simulink model "plataforma_unlp_GSAFE_v2"  (R2016b)
settings: Solver=ode1  StartTime=escenario.ti  StopTime=escenario.tf  FixedStep=escenario.paso  RelTol=1e-3  EnableMultiTasking=on
undefined symbols (not defined in the file): ctrl, escenario, hardware, lazo, lazoh, parametros, PDB_IFB_GSAFE_v2, settings
settings Model: Creator=Administrador  LastModifiedBy=Nicolas
settings DataIOCC: SaveFormat=Array  SaveState=on  StateSaveName=estados  OutputSaveName=salidas
settings OptimizationCC: ExpressionDepthLimit=2147483647  LifeSpan=inf
settings DebuggingCC: UnderspecifiedInitializationDetection=Classic  MergeDetectMultiDrivingBlocksExec=none  SolverPrmCheckMsg=warning  StateNameClashWarn=warning  SFUnexpectedBacktrackingDiag=warning  SFNoUnconditionalDefaultTransitionDiag=warning  SFExecutionAtInitializationDiag=none
settings HardwareCC: ProdBitPerPointer=32  ProdBitPerSizeT=32  ProdBitPerPtrDiffT=32  ProdLargestAtomicFloat=None  ProdIntDivRoundTo=Undefined  ProdEndianess=Unspecified  ProdWordSize=32  ProdHWDeviceType=32-bit Generic
settings ModelReferenceCC: PropagateSignalLabelsOutOfModel=off
settings GRTTargetCC: TargetLangStandard=C89/C90 (ANSI)  GeneratePreprocessorConditionals=Disable all
settings ConfigComp: CovMetricSettings=dw  CovHtmlReporting=on  CovSaveCumulativeToWorkspaceVar=on  CovSaveSingleToWorkspaceVar=on  CovExternalEMLEnable=off

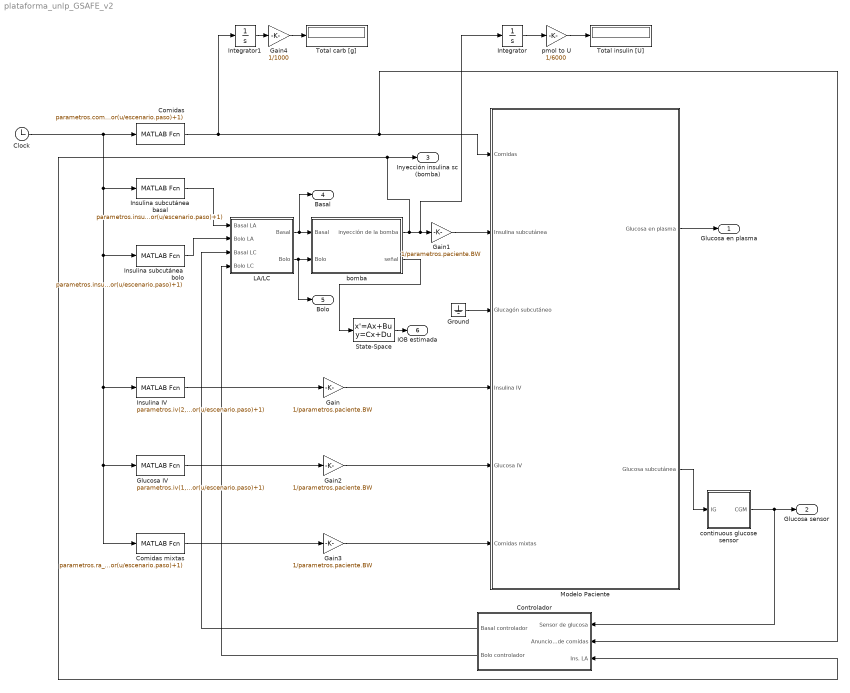
== system plataforma_unlp_GSAFE_v2 ==
  Clock : Clock
  Comidas : MATLABFcn  MATLABFcn=parametros.comidas(1,floor(u/escenario.paso)+1)  OutputDimensions=1  OutputSignalType=real  Output1D=off
  Comidas mixtas : MATLABFcn  MATLABFcn=parametros.ra_comidas_mixtas(1,floor(u/escenario.paso)+1)  OutputDimensions=1  OutputSignalType=real  Output1D=off
  Controlador : Subsystem
  Gain{,1..3} (4 alike) : Gain  Gain=1/parametros.paciente.BW
  Gain4 : Gain  Gain=1/1000
  Glucosa IV : MATLABFcn  MATLABFcn=parametros.iv(1,floor(u/escenario.paso)+1)  OutputDimensions=1  OutputSignalType=real  Output1D=off
  Ground : Ground
  Insulina IV : MATLABFcn  MATLABFcn=parametros.iv(2,floor(u/escenario.paso)+1)  OutputDimensions=1  OutputSignalType=real  Output1D=off
  Insulina subcutánea basal : MATLABFcn  MATLABFcn=parametros.insulina(2,floor(u/escenario.paso)+1)  OutputDimensions=1  OutputSignalType=real  Output1D=off
  Insulina subcutánea bolo : MATLABFcn  MATLABFcn=parametros.insulina(1,floor(u/escenario.paso)+1)  OutputDimensions=1  OutputSignalType=real  Output1D=off
  Integrator : Integrator
  Integrator1 : Integrator
  LA/LC : Subsystem
  Modelo Paciente : Subsystem
  State-Space : StateSpace  A=[-ctrl.KDIA 0;ctrl.KDIA -ctrl.KDIA]  B=[1/6000;0]  C=[1 1]  D=0  X0=[ctrl.Iee/ctrl.KDIA/6000;ctrl.Iee/ctrl.KDIA/6000]
  Total carb [g] : Display
  Total insulin [U] : Display
  bomba : Subsystem
  continuous glucose sensor : Subsystem
  pmol to U : Gain  Gain=1/6000
  Glucosa en plasma : Outport
  Glucosa sensor : Outport  Port=2
  Inyección insulina sc (bomba) : Outport  Port=3
  Basal : Outport  Port=4
  Bolo : Outport  Port=5
  IOB estimada : Outport  Port=6
  wires:
  Insulina IV/1 -> Gain/1
  Gain/1 -> Modelo Paciente/4(Insulina IV)
  Gain1/1 -> Modelo Paciente/2(Insulina subcutánea)
  Glucosa IV/1 -> Gain2/1
  Gain2/1 -> Modelo Paciente/5(Glucosa IV)
  Comidas/1 -> Integrator1/1, Controlador/2(Anuncio de comidas), Modelo Paciente/1(Comidas)
  Comidas mixtas/1 -> Gain3/1
  Gain3/1 -> Modelo Paciente/6(Comidas mixtas)
  Modelo Paciente/2(Glucosa subcutánea) -> continuous glucose sensor/1(IG)
  continuous glucose sensor/1(CGM) -> Glucosa sensor/1, Controlador/1(Sensor de glucosa)
  bomba/1(inyección de la bomba) -> Controlador/3(Ins. LA), Inyección insulina sc (bomba)/1, Integrator/1, Gain1/1
  bomba/2(señal) -> State-Space/1
  Insulina subcutánea basal/1 -> LA/LC/1(Basal LA)
  Insulina subcutánea bolo/1 -> LA/LC/2(Bolo LA)
  Controlador/1(Basal controlador) -> LA/LC/3(Basal LC)
  Controlador/2(Bolo controlador) -> LA/LC/4(Bolo LC)
  LA/LC/1(Basal) -> Basal/1, bomba/1(Basal)
  LA/LC/2(Bolo) -> bomba/2(Bolo), Bolo/1
  Integrator1/1 -> Gain4/1
  Gain4/1 -> Total carb [g]/1
  Integrator/1 -> pmol to U/1
  pmol to U/1 -> Total insulin [U]/1
  Clock/1 -> Comidas/1, Insulina subcutánea bolo/1, Comidas mixtas/1, Glucosa IV/1, Insulina IV/1, Insulina subcutánea basal/1
  State-Space/1 -> IOB estimada/1
  Modelo Paciente/1(Glucosa en plasma) -> Glucosa en plasma/1
  Ground/1 -> Modelo Paciente/3(Glucagón subcutáneo)

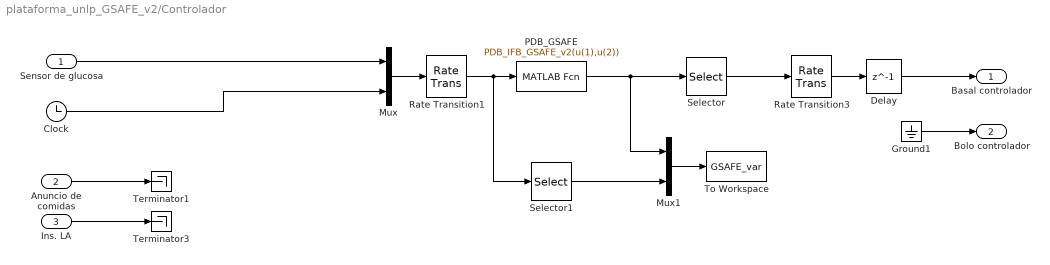
== system plataforma_unlp_GSAFE_v2/Controlador ==
  Sensor de glucosa : Inport
  Anuncio de comidas : Inport  Port=2
  Ins. LA : Inport  Port=3
  Clock : Clock
  Delay : Delay  DelayLength=1  InitialCondition=ctrl.Iee  SampleTime=ctrl.paso
  Ground1 : Ground
  Mux : Mux  Inputs=2
  Mux1 : Mux  Inputs=2
  PDB_GSAFE : MATLABFcn  MATLABFcn=PDB_IFB_GSAFE_v2(u(1),u(2))  OutputDimensions=2
  Rate Transition1 : RateTransition  OutPortSampleTime=ctrl.Ts
  Rate Transition3 : RateTransition  X0=ctrl.Iee  OutPortSampleTime=ctrl.paso
  Selector : Selector  InputPortWidth=2  IndexOptions=Index vector (dialog)  Indices=1  OutputSizes=1
  Selector1 : Selector  InputPortWidth=2  IndexOptions=Index vector (dialog)  Indices=1  OutputSizes=1
  Terminator1 : Terminator
  Terminator3 : Terminator
  To Workspace : ToWorkspace  VariableName=GSAFE_var  SampleTime=ctrl.Ts
  Basal controlador : Outport
  Bolo controlador : Outport  Port=2
  wires:
  Ins. LA/1 -> Terminator3/1
  Mux/1 -> Rate Transition1/1
  PDB_GSAFE/1 -> Mux1/1, Selector/1
  Ground1/1 -> Bolo controlador/1
  Rate Transition3/1 -> Delay/1
  Selector/1 -> Rate Transition3/1
  Mux1/1 -> To Workspace/1
  Sensor de glucosa/1 -> Mux/1
  Anuncio de comidas/1 -> Terminator1/1
  Rate Transition1/1 -> Selector1/1, PDB_GSAFE/1
  Clock/1 -> Mux/2
  Selector1/1 -> Mux1/2
  Delay/1 -> Basal controlador/1

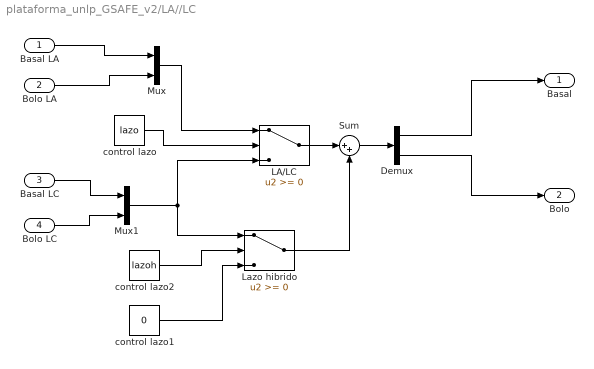
== system plataforma_unlp_GSAFE_v2/LA//LC ==
  Basal LA : Inport
  Bolo LA : Inport  Port=2
  Basal LC : Inport  Port=3
  Bolo LC : Inport  Port=4
  Demux : Demux  Outputs=2
  LA/LC : Switch
  Lazo hibrido : Switch
  Mux : Mux  Inputs=2
  Mux1 : Mux  Inputs=2
  Sum : Sum  Inputs=|++
  control lazo : Constant  Value=lazo
  control lazo1 : Constant  Value=0
  control lazo2 : Constant  Value=lazoh
  Basal : Outport
  Bolo : Outport  Port=2
  wires:
  Basal LA/1 -> Mux/1
  Bolo LA/1 -> Mux/2
  Basal LC/1 -> Mux1/1
  Bolo LC/1 -> Mux1/2
  Mux/1 -> LA/LC/1
  control lazo/1 -> LA/LC/2
  Mux1/1 -> LA/LC/3, Lazo hibrido/1
  Demux/1 -> Basal/1
  Demux/2 -> Bolo/1
  LA/LC/1 -> Sum/1
  Sum/1 -> Demux/1
  Lazo hibrido/1 -> Sum/2
  control lazo2/1 -> Lazo hibrido/2
  control lazo1/1 -> Lazo hibrido/3

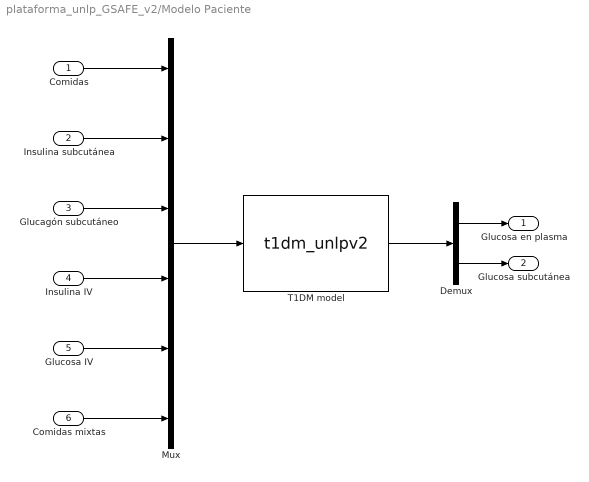
== system plataforma_unlp_GSAFE_v2/Modelo Paciente ==
  Comidas : Inport
  Insulina subcutánea : Inport  Port=2
  Glucagón subcutáneo : Inport  Port=3
  Insulina IV : Inport  Port=4
  Glucosa IV : Inport  Port=5
  Comidas mixtas : Inport  Port=6
  Demux : Demux  Outputs=2
  Mux : Mux  Inputs=6
  T1DM model : S-Function  FunctionName=t1dm_unlpv2  Parameters=parametros,escenario  SFunctionDeploymentMode=off  EnableBusSupport=off
  Glucosa en plasma : Outport
  Glucosa subcutánea : Outport  Port=2
  wires:
  Mux/1 -> T1DM model/1
  Insulina subcutánea/1 -> Mux/2
  Insulina IV/1 -> Mux/4
  Glucosa IV/1 -> Mux/5
  Comidas/1 -> Mux/1
  Comidas mixtas/1 -> Mux/6
  T1DM model/1 -> Demux/1
  Glucagón subcutáneo/1 -> Mux/3
  Demux/1 -> Glucosa en plasma/1
  Demux/2 -> Glucosa subcutánea/1

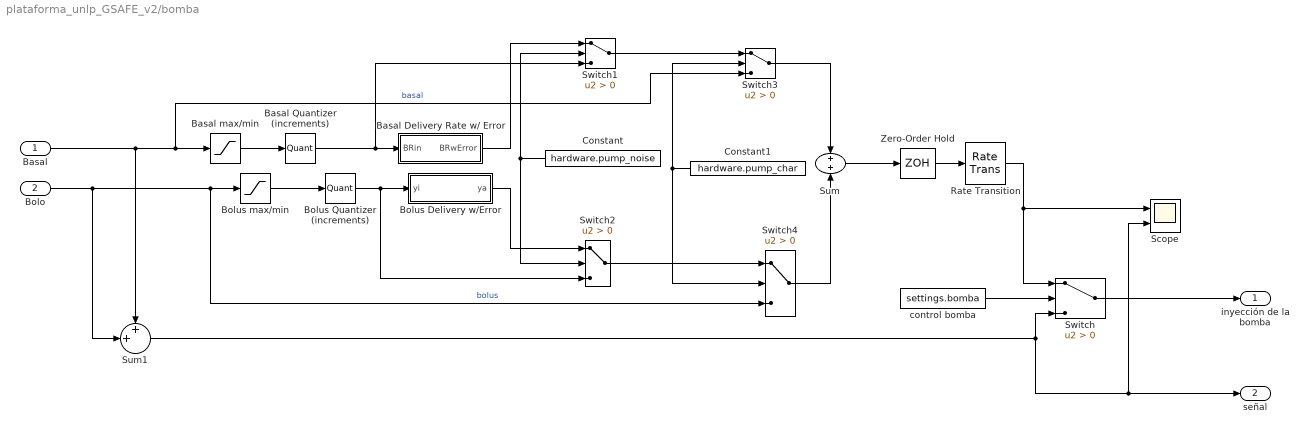
== system plataforma_unlp_GSAFE_v2/bomba ==
  Basal : Inport
  Bolo : Inport  Port=2
  Basal Delivery Rate w/ Error : Subsystem
  Basal Quantizer (increments) : Quantizer  QuantizationInterval=hardware.pump_basal_inc
  Basal max/min : Saturate  UpperLimit=hardware.pump_basal_max  LowerLimit=hardware.pump_basal_min
  Bolus Delivery w/Error : Subsystem
  Bolus Quantizer (increments) : Quantizer  QuantizationInterval=hardware.pump_bolus_inc
  Bolus max/min : Saturate  UpperLimit=hardware.pump_bolus_max  LowerLimit=0
  Constant : Constant  Value=hardware.pump_noise
  Constant1 : Constant  Value=hardware.pump_char
  Rate Transition : RateTransition
  Scope : Scope  NumInputPorts=2
  Sum : Sum  Inputs=+|+
  Sum1 : Sum  Inputs=++|
  Switch{,1..4} (5 alike) : Switch  Criteria=u2 > Threshold
  Zero-Order Hold : ZeroOrderHold  SampleTime=hardware.pump_sampling
  control bomba : Constant  Value=settings.bomba
  inyección de la bomba : Outport
  señal : Outport  Port=2
  wires:
  control bomba/1 -> Switch/2
  Switch/1 -> inyección de la bomba/1
  Sum1/1 -> Scope/2, señal/1, Switch/3
  Zero-Order Hold/1 -> Rate Transition/1
  Bolus max/min/1 -> Bolus Quantizer (increments)/1
  Sum/1 -> Zero-Order Hold/1
  Basal/1 -> Sum1/1, Basal max/min/1, Switch3/3  "basal"
  Basal max/min/1 -> Basal Quantizer (increments)/1
  Bolo/1 -> Sum1/2, Switch4/3, Bolus max/min/1  "bolus"
  Bolus Quantizer (increments)/1 -> Switch2/3, Bolus Delivery w/Error/1(yi)
  Basal Quantizer (increments)/1 -> Switch1/3, Basal Delivery Rate w/ Error/1(BRin)
  Basal Delivery Rate w/ Error/1(BRwError) -> Switch1/1
  Constant/1 -> Switch2/2, Switch1/2
  Bolus Delivery w/Error/1(ya) -> Switch2/1
  Switch2/1 -> Switch4/1
  Switch1/1 -> Switch3/1
  Constant1/1 -> Switch4/2, Switch3/2
  Switch3/1 -> Sum/1
  Switch4/1 -> Sum/2
  Rate Transition/1 -> Scope/1, Switch/1

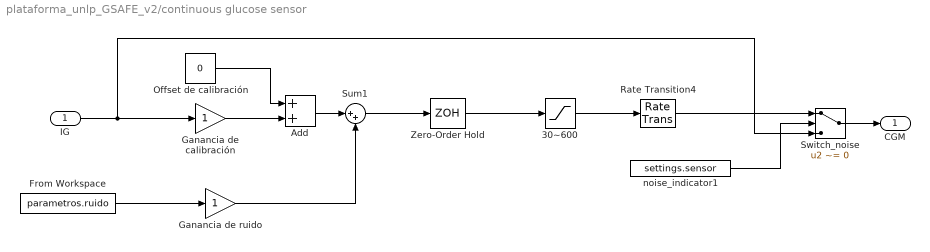
== system plataforma_unlp_GSAFE_v2/continuous glucose sensor ==
  IG : Inport
  30~600 : Saturate  UpperLimit=hardware.sensor_max  LowerLimit=hardware.sensor_min
  Add : Sum
  From Workspace : FromWorkspace  VariableName=parametros.ruido  SampleTime=0
  Ganancia de calibración : Gain
  Ganancia de ruido : Gain
  Offset de calibración : Constant  Value=0
  Rate Transition4 : RateTransition  X0=parametros.paciente.x0(4)/parametros.paciente.Vg  OutPortSampleTime=escenario.paso
  Sum1 : Sum  Inputs=|++
  Switch_noise : Switch  Criteria=u2 ~= 0  Threshold=1440
  Zero-Order Hold : ZeroOrderHold  SampleTime=hardware.sensor_sampling
  noise_indicator1 : Constant  Value=settings.sensor
  CGM : Outport
  wires:
  Sum1/1 -> Zero-Order Hold/1
  Zero-Order Hold/1 -> 30~600/1
  30~600/1 -> Rate Transition4/1
  Offset de calibración/1 -> Add/1
  Ganancia de calibración/1 -> Add/2
  Add/1 -> Sum1/1
  Rate Transition4/1 -> Switch_noise/1
  noise_indicator1/1 -> Switch_noise/2
  IG/1 -> Switch_noise/3, Ganancia de calibración/1
  Switch_noise/1 -> CGM/1
  From Workspace/1 -> Ganancia de ruido/1
  Ganancia de ruido/1 -> Sum1/2

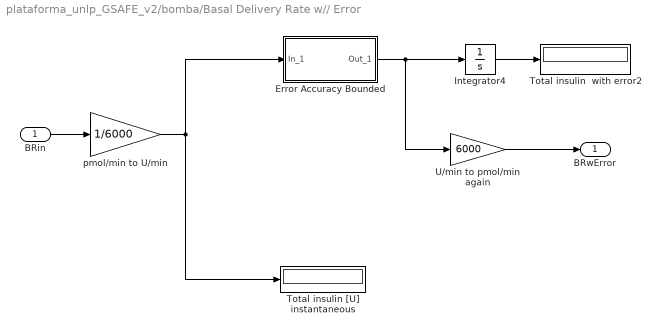
== system plataforma_unlp_GSAFE_v2/bomba/Basal Delivery Rate w// Error ==
  BRin : Inport
  Error Accuracy Bounded : Subsystem
  Integrator4 : Integrator
  Total insulin  with error2 : Display
  Total insulin [U] instantaneous : Display
  U/min to pmol/min again : Gain  Gain=6000
  pmol/min to U/min : Gain  Gain=1/6000
  BRwError : Outport
  wires:
  Integrator4/1 -> Total insulin  with error2/1
  Error Accuracy Bounded/1(Out_1) -> Integrator4/1, U/min to pmol/min again/1
  U/min to pmol/min again/1 -> BRwError/1
  pmol/min to U/min/1 -> Error Accuracy Bounded/1(In_1), Total insulin [U] instantaneous/1
  BRin/1 -> pmol/min to U/min/1

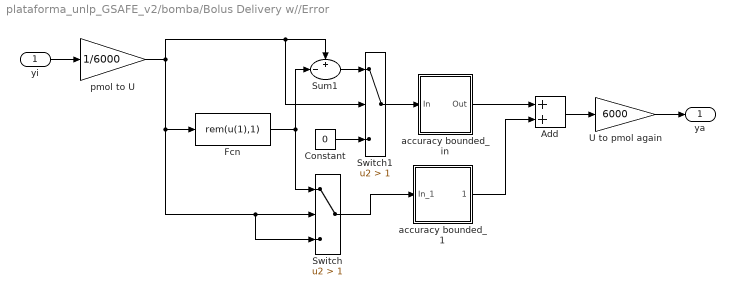
== system plataforma_unlp_GSAFE_v2/bomba/Bolus Delivery w//Error ==
  yi : Inport
  Add : Sum
  Constant : Constant  Value=0
  Fcn : Fcn  Expr=rem(u(1),1)
  Sum1 : Sum  Inputs=+-|
  Switch : Switch  Criteria=u2 > Threshold  Threshold=1
  Switch1 : Switch  Criteria=u2 > Threshold  Threshold=1
  U to pmol again : Gain  Gain=6000
  accuracy bounded_1 : Subsystem
  accuracy bounded_in : Subsystem
  pmol to U : Gain  Gain=1/6000
  ya : Outport
  wires:
  Switch1/1 -> accuracy bounded_in/1(In)
  Constant/1 -> Switch1/3
  Sum1/1 -> Switch1/1
  Switch/1 -> accuracy bounded_1/1(In_1)
  Fcn/1 -> Sum1/2, Switch/1
  accuracy bounded_1/1(Out_1) -> Add/2
  accuracy bounded_in/1(Out) -> Add/1
  Add/1 -> U to pmol again/1
  U to pmol again/1 -> ya/1
  pmol to U/1 -> Switch1/2, Sum1/1, Switch/3, Switch/2, Fcn/1
  yi/1 -> pmol to U/1

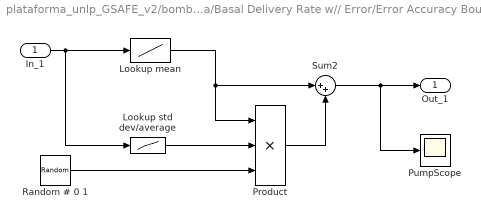
== system plataforma_unlp_GSAFE_v2/bomba/Basal Delivery Rate w// Error/Error Accuracy Bounded ==
  In_1 : Inport
  Lookup mean : Lookup  InputValues=hardware.pump_accuracy_bolus_amount  Table=hardware.pump_bolus_mean
  Lookup std dev/average : Lookup  InputValues=hardware.pump_accuracy_bolus_amount  Table=hardware.pump_bolus_std2
  Product : Product  Inputs=3  RndMeth=Zero
  PumpScope : Scope
  "Random # 0 1 " : RandomNumber  SampleTime=escenario.paso
  Sum2 : Sum  Inputs=|++
  Out_1 : Outport
  wires:
  In_1/1 -> Lookup std dev/average/1, Lookup mean/1
  "Random # 0 1 "/1 -> Product/3
  Lookup std dev/average/1 -> Product/2
  Product/1 -> Sum2/2
  Sum2/1 -> Out_1/1, PumpScope/1
  Lookup mean/1 -> Sum2/1, Product/1

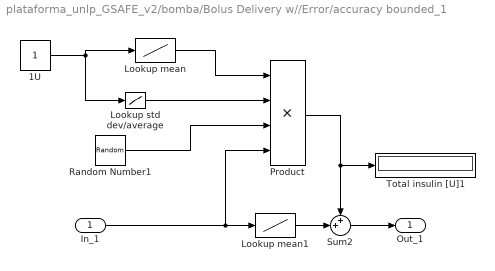
== system plataforma_unlp_GSAFE_v2/bomba/Bolus Delivery w//Error/accuracy bounded_1 ==
  In_1 : Inport
  1U : Constant
  Lookup mean : Lookup  InputValues=hardware.pump_accuracy_bolus_amount  Table=hardware.pump_bolus_mean  LookUpMeth=Interpolation-Use End Values
  Lookup mean1 : Lookup  InputValues=hardware.pump_accuracy_bolus_amount  Table=hardware.pump_bolus_mean
  Lookup std dev/average : Lookup  InputValues=hardware.pump_accuracy_bolus_amount  Table=hardware.pump_bolus_std2  LookUpMeth=Interpolation-Use End Values
  Product : Product  Inputs=4  RndMeth=Zero
  Random Number1 : RandomNumber  SampleTime=escenario.paso
  Sum2 : Sum  Inputs=++|
  Total insulin [U]1 : Display
  Out_1 : Outport
  wires:
  Product/1 -> Total insulin [U]1/1, Sum2/1
  Lookup mean1/1 -> Sum2/2
  In_1/1 -> Lookup mean1/1, Product/4
  1U/1 -> Lookup std dev/average/1, Lookup mean/1
  Sum2/1 -> Out_1/1
  Random Number1/1 -> Product/3
  Lookup std dev/average/1 -> Product/2
  Lookup mean/1 -> Product/1

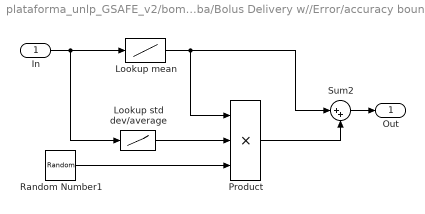
== system plataforma_unlp_GSAFE_v2/bomba/Bolus Delivery w//Error/accuracy bounded_in ==
  In : Inport
  Lookup mean : Lookup  InputValues=hardware.pump_accuracy_bolus_amount  Table=hardware.pump_bolus_mean
  Lookup std dev/average : Lookup  InputValues=hardware.pump_accuracy_bolus_amount  Table=hardware.pump_bolus_std2  LookUpMeth=Interpolation-Use End Values
  Product : Product  Inputs=3  RndMeth=Zero
  Random Number1 : RandomNumber  SampleTime=escenario.paso
  Sum2 : Sum  Inputs=|++
  Out : Outport
  wires:
  Sum2/1 -> Out/1
  In/1 -> Lookup mean/1, Lookup std dev/average/1
  Product/1 -> Sum2/2
  Lookup mean/1 -> Sum2/1, Product/1
  Random Number1/1 -> Product/3
  Lookup std dev/average/1 -> Product/2
